simulink model "STDiscovery"  (R2017b)
settings: Solver=FixedStepAuto  StartTime=0.0  StopTime=0.01  FixedStep=Abtastzeit  RelTol=1e-3
PreLoadFcn:
  | waijung.modelPreload; % Required for working with Waijung Blockset. Do not remove.
model workspace (MAT data in the model file):
  Abtastzeit = 0.01
  Servo_IN_min = 0.894
  SimulationDutyCycle = 27
undefined symbols (not defined in the file): HSEOSC, Link, LQFP176, ST, Statusbits, Steuerbits, STM32F417IG
libraries: simulink x17, stm32f4_io_lib x16, simulink_extras x8, stm32f4_adc_lib x7, powerlib_meascontrol x4, stm32f4_device_config_lib x1
(part 4 of 4)

== system STDiscovery/Aktorik/Ansteuerung Motor/Skaliere PWM Ausgang wieder in wert zwischen( + -100) zum Loggen  ==
  note: in muss immer mit kleinstem wert anfangen
  note: 100(Gas)
      | -100(Rückwärts)
  note: %
  Wert in % für 50Hz PWM : Inport
  Constant1 : Constant  Value=100
  Constant2 : Constant  Value=0
  Constant3 : Constant  Value=-100
  Constant4 : Constant  Value=5.5
  Constant5 : Constant  Value=7.45
  Constant6 : Constant  Value=9.5
  Skaliere lN nach OUT : Subsystem
  "Wert zwischen 100 und -100 " : Outport
  wires:
  Skaliere lN nach OUT/1(OUT_SIGNAL) -> "Wert zwischen 100 und -100 "/1
  Wert in % für 50Hz PWM/1 -> Skaliere lN nach OUT/1(IN_SIGNAL)
  Constant1/1 -> Skaliere lN nach OUT/5(OUT_min)
  Constant2/1 -> Skaliere lN nach OUT/6(OUT_mitte)
  Constant3/1 -> Skaliere lN nach OUT/7(OUT_max)
  Constant6/1 -> Skaliere lN nach OUT/4(IN_max)
  Constant5/1 -> Skaliere lN nach OUT/3(IN_mitte)
  Constant4/1 -> Skaliere lN nach OUT/2(IN_min)

== system STDiscovery/Aktorik/Ansteuerung Servo/Logik  ==
  Fernbedienung Signal : Inport
  Moduswahl (1=autonom 0=manuell) : Inport  Port=2
  Jetson Signal : Inport  Port=3
  "(Einschaltverzögerung) Wartezeit Anhalten Erst 1s aktuellen autonomen Lenkeinschlag halten, dann Fernbedienung übernehmen " : powerlib_meascontrol/Logic/On Delay  DelayType=On delay  delay=1  ic=1  Ts=0
      settings: SourceProductName=Simscape Power Systems
  Data Type Conversion : DataTypeConversion  OutDataTypeStr=double
  "Erst 1s aktuellen autonomen Lenkeinschlag halten, dann Fernbedienung übernehmen" : Switch  Criteria=u2 > Threshold
  Modus Auswahl : Switch  Criteria=u2 > Threshold
  Output Pin : Outport
  wires:
  Data Type Conversion/1 -> "Erst 1s aktuellen autonomen Lenkeinschlag halten, dann Fernbedienung übernehmen"/3  "manuell"
  Moduswahl (1=autonom 0=manuell)/1 -> "(Einschaltverzögerung) Wartezeit Anhalten Erst 1s aktuellen autonomen Lenkeinschlag halten, dann Fernbedienung übernehmen "/1, Modus Auswahl/2
  Modus Auswahl/1 -> Output Pin/1  "Ausgang zum servo"
  "Erst 1s aktuellen autonomen Lenkeinschlag halten, dann Fernbedienung übernehmen"/1 -> Modus Auswahl/3  "manuell"
  Jetson Signal/1 -> Modus Auswahl/1, "Erst 1s aktuellen autonomen Lenkeinschlag halten, dann Fernbedienung übernehmen"/1  "autonom"
  "(Einschaltverzögerung) Wartezeit Anhalten Erst 1s aktuellen autonomen Lenkeinschlag halten, dann Fernbedienung übernehmen "/1 -> "Erst 1s aktuellen autonomen Lenkeinschlag halten, dann Fernbedienung übernehmen"/2
  Fernbedienung Signal/1 -> Data Type Conversion/1

== system STDiscovery/Aktorik/Ansteuerung Servo/Plausibilitäts Check ==
  In1 : Inport
  "Gib Mittelstellung aus, wenn mit Signal etwas nicht Stimmt" : Switch  Criteria=u2 > Threshold
  Logical Operator : Logic  AllPortsSameDT=off  OutDataTypeStr=boolean
  Mittelstellung : Constant  Value=0.001407
  Relational Operator : RelationalOperator  Operator=<  OutDataTypeStr=boolean  RndMeth=Nearest
  Relational Operator1 : RelationalOperator  Operator=>  OutDataTypeStr=boolean  RndMeth=Nearest
  "ok max " : Constant  Value=0.0021
  ok min : Constant  Value=0.0008
  Out1 : Outport
  wires:
  In1/1 -> Relational Operator1/1, Relational Operator/1, "Gib Mittelstellung aus, wenn mit Signal etwas nicht Stimmt"/1
  Logical Operator/1 -> "Gib Mittelstellung aus, wenn mit Signal etwas nicht Stimmt"/2
  "Gib Mittelstellung aus, wenn mit Signal etwas nicht Stimmt"/1 -> Out1/1
  Mittelstellung/1 -> "Gib Mittelstellung aus, wenn mit Signal etwas nicht Stimmt"/3
  Relational Operator1/1 -> Logical Operator/2
  Relational Operator/1 -> Logical Operator/1
  ok min/1 -> Relational Operator1/2
  "ok max "/1 -> Relational Operator/2

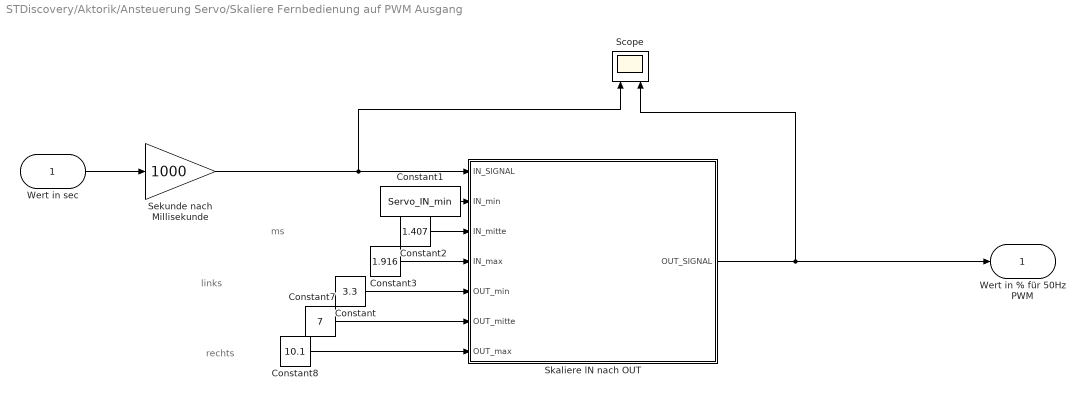
== system STDiscovery/Aktorik/Ansteuerung Servo/Skaliere Fernbedienung auf PWM Ausgang ==
  note: ms
  note: links
  note: rechts
  Wert in sec : Inport
  Constant : Constant  Value=3.3
  Constant1 : Constant  Value=Servo_IN_min
  Constant2 : Constant  Value=1.407
  Constant3 : Constant  Value=1.916
  Constant7 : Constant  Value=7
  Constant8 : Constant  Value=10.1
  Scope : Scope  NumInputPorts=2
  Sekunde nach Millisekunde : Gain  Gain=1000
  Skaliere lN nach OUT : Subsystem
  Wert in % für 50Hz PWM : Outport
  wires:
  Constant/1 -> Skaliere lN nach OUT/5(OUT_min)
  Wert in sec/1 -> Sekunde nach Millisekunde/1
  Skaliere lN nach OUT/1(OUT_SIGNAL) -> Scope/2, Wert in % für 50Hz PWM/1
  Constant3/1 -> Skaliere lN nach OUT/4(IN_max)
  Constant2/1 -> Skaliere lN nach OUT/3(IN_mitte)
  Constant1/1 -> Skaliere lN nach OUT/2(IN_min)
  Sekunde nach Millisekunde/1 -> Scope/1, Skaliere lN nach OUT/1(IN_SIGNAL)
  Constant7/1 -> Skaliere lN nach OUT/6(OUT_mitte)
  Constant8/1 -> Skaliere lN nach OUT/7(OUT_max)

== system STDiscovery/Aktorik/Ansteuerung Servo/Skaliere Stellwinkel auf PWM Ausgang ==
  note: Stellwinkel
  note: rechts
  note: links
  Stellwinkel : Inport
  Constant : Constant  Value=3.3
  Constant1 : Constant  Value=-25
  Constant2 : Constant  Value=0
  Constant3 : Constant  Value=25
  Constant7 : Constant  Value=7
  Constant8 : Constant  Value=10.1
  Skaliere lN nach OUT : Subsystem
  Wert in % für 50Hz PWM : Outport
  wires:
  Constant/1 -> Skaliere lN nach OUT/5(OUT_min)
  Skaliere lN nach OUT/1(OUT_SIGNAL) -> Wert in % für 50Hz PWM/1
  Constant3/1 -> Skaliere lN nach OUT/4(IN_max)
  Constant2/1 -> Skaliere lN nach OUT/3(IN_mitte)
  Constant1/1 -> Skaliere lN nach OUT/2(IN_min)
  Stellwinkel/1 -> Skaliere lN nach OUT/1(IN_SIGNAL)
  Constant8/1 -> Skaliere lN nach OUT/7(OUT_max)
  Constant7/1 -> Skaliere lN nach OUT/6(OUT_mitte)

== system STDiscovery/Aktorik/Ansteuerung Servo/Skaliere steuer Stellwinkel wieder in Grad zum Loggen ==
  note: rechts
  note: links
  note: Stellwinkel
  Wert in % für 50Hz PWM : Inport
  Constant : Constant  Value=3.3
  Constant1 : Constant  Value=-25
  Constant2 : Constant  Value=0
  Constant3 : Constant  Value=25
  Constant7 : Constant  Value=7
  Constant8 : Constant  Value=10.1
  Skaliere lN nach OUT : Subsystem
  Stellwinkel : Outport
  wires:
  Skaliere lN nach OUT/1(OUT_SIGNAL) -> Stellwinkel/1
  Constant/1 -> Skaliere lN nach OUT/2(IN_min)
  Wert in % für 50Hz PWM/1 -> Skaliere lN nach OUT/1(IN_SIGNAL)
  Constant7/1 -> Skaliere lN nach OUT/3(IN_mitte)
  Constant8/1 -> Skaliere lN nach OUT/4(IN_max)
  Constant2/1 -> Skaliere lN nach OUT/6(OUT_mitte)
  Constant3/1 -> Skaliere lN nach OUT/7(OUT_max)
  Constant1/1 -> Skaliere lN nach OUT/5(OUT_min)

== system STDiscovery/Aktorik/Modusauswahl Autonom oder Manuell Ueberwachung ob Eingriff durch Fernbedienung/Motor Überwachung Eingriff durch Fernbedienung? ==
  Dutycycle in % : Inport
  Betrag bilden für negative Abweichunge : Abs
  Ist die Aktuelle Abweichung größer als die Maximal erlaubte? : RelationalOperator  Operator=>  OutDataTypeStr=boolean  RndMeth=Nearest
  Maximale Abweichung : Constant  Value=0.2
  "Mittelwert, in % wenn Fernsteuerung in der Mitte steht" : Constant  Value=7.45
  Subtract : Sum  Inputs=|+-
  Ja/Nein : Outport
  wires:
  "Mittelwert, in % wenn Fernsteuerung in der Mitte steht"/1 -> Subtract/2
  Betrag bilden für negative Abweichunge/1 -> Ist die Aktuelle Abweichung größer als die Maximal erlaubte?/1
  Maximale Abweichung/1 -> Ist die Aktuelle Abweichung größer als die Maximal erlaubte?/2
  Dutycycle in %/1 -> Subtract/1
  Subtract/1 -> Betrag bilden für negative Abweichunge/1
  Ist die Aktuelle Abweichung größer als die Maximal erlaubte?/1 -> Ja/Nein/1

== system STDiscovery/Aktorik/Modusauswahl Autonom oder Manuell Ueberwachung ob Eingriff durch Fernbedienung/Servo Überwachung Eingriff durch Fernbedienung? ==
  Dutycycle in % : Inport
  Betrag bilden für negative Abweichungen : Abs
  Ist die aktuelle Abweichung größer als die maximal erlaubte? : RelationalOperator  Operator=>  OutDataTypeStr=boolean  RndMeth=Nearest
  Maximale Abweichung : Constant  Value=0.2
  "Mittelwert, in % wenn Fernsteuerung in der Mitte steht" : Constant  Value=7
  Subtract : Sum  Inputs=|+-
  Ja/Nein : Outport
  wires:
  "Mittelwert, in % wenn Fernsteuerung in der Mitte steht"/1 -> Subtract/2
  Betrag bilden für negative Abweichungen/1 -> Ist die aktuelle Abweichung größer als die maximal erlaubte?/1
  Maximale Abweichung/1 -> Ist die aktuelle Abweichung größer als die maximal erlaubte?/2
  Dutycycle in %/1 -> Subtract/1
  Subtract/1 -> Betrag bilden für negative Abweichungen/1
  Ist die aktuelle Abweichung größer als die maximal erlaubte?/1 -> Ja/Nein/1

== system STDiscovery/Debug/Subsystem/Safety 2.5 |<--->|12.5 ==
  In1 : Inport
  Constant : Constant  Value=2.5
  Constant1 : Constant  Value=12.5
  Data Type Conversion : DataTypeConversion
  Data Type Conversion1 : DataTypeConversion
  Switch : Switch  Criteria=u2 > Threshold  Threshold=2.5
  Switch1 : Switch  Criteria=u2 > Threshold  Threshold=12.5
  Out1 : Outport
  wires:
  Switch/1 -> Switch1/3, Switch1/2
  In1/1 -> Switch/1, Switch/2
  Switch1/1 -> Out1/1
  Constant/1 -> Data Type Conversion/1
  Constant1/1 -> Data Type Conversion1/1
  Data Type Conversion1/1 -> Switch1/1
  Data Type Conversion/1 -> Switch/3

== system STDiscovery/Debug/Subsystem1/Safety 2.5 |<--->|12.5 ==
  In1 : Inport
  Constant : Constant  Value=2.5
  Constant1 : Constant  Value=12.5
  Data Type Conversion : DataTypeConversion
  Data Type Conversion1 : DataTypeConversion
  Switch : Switch  Criteria=u2 > Threshold  Threshold=2.5
  Switch1 : Switch  Criteria=u2 > Threshold  Threshold=12.5
  Out1 : Outport
  wires:
  Switch/1 -> Switch1/3, Switch1/2
  In1/1 -> Switch/1, Switch/2
  Switch1/1 -> Out1/1
  Constant/1 -> Data Type Conversion/1
  Constant1/1 -> Data Type Conversion1/1
  Data Type Conversion1/1 -> Switch1/1
  Data Type Conversion/1 -> Switch/3

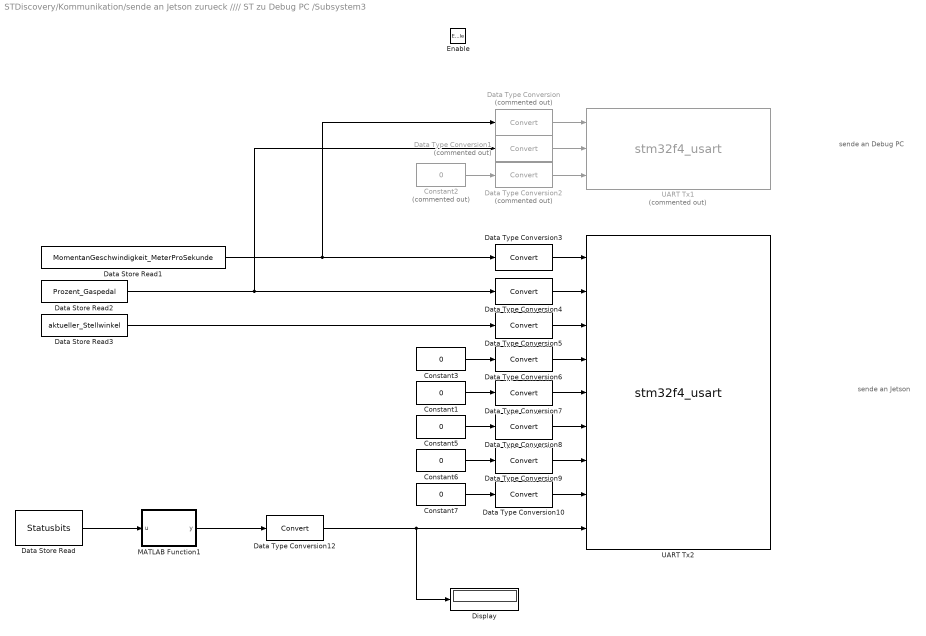
== system STDiscovery/Kommunikation/sende an Jetson zurueck //// ST zu Debug PC /Subsystem3 ==
  note: sende an Debug PC
  note: sende an Jetson
  Enable : EnablePort
  Constant{1,3,5..7} (5 alike) : Constant  Value=0
  Constant2 : Constant  Commented=on  Value=0
  Data Store Read : DataStoreRead  DataStoreName=Statusbits
  Data Store Read1 : DataStoreRead  DataStoreName=MomentanGeschwindigkeit_MeterProSekunde
  Data Store Read2 : DataStoreRead  DataStoreName=Prozent_Gaspedal
  Data Store Read3 : DataStoreRead  DataStoreName=aktueller_Stellwinkel
  Data Type Conversion : DataTypeConversion  Commented=on
  Data Type Conversion1 : DataTypeConversion  Commented=on
  Data Type Conversion{3..10,12} (9 alike) : DataTypeConversion
  Data Type Conversion2 : DataTypeConversion  Commented=on
  Display : Display
  MATLAB Function1 : MATLAB Function  TreatAsAtomicUnit=on
  UART Tx1 : S-Function  Priority=1  Commented=on  FunctionName=stm32f4_usart  Parameters=configuration,uartmodule,transfer,baudrate,inputtype,outputtype,confstr,binheaderarray,binterminatorarray,asciiheader,asciiterminator,bindatalength,packetmode,varname,sampletime,sampletimestr,blockid  SFunctionDeploymentMode=off  EnableBusSupport=off  mask(stm32f4_usart){configuration=Tx, uartmodule=3, baudrate=115200, databits=8, parity=No, stopbit=1, remaptxpin=Not used, remaprxpin=Not used, flowcontrol=None, remapctspin=Not used, remaprtspin=Not used, advanceoptions=off, rxbuffersize=512, txbuffersize=512, transfer=Blocking, packetmode=Ascii, binheader='7E 7E', binterminator='03 03', porttype_double=1, porttype_single=0, porttype_int8=1, porttype_uint8=0, porttype_int16=0, porttype_uint16=0, porttype_int32=0, porttype_uint32=0, asciiformat='Antwort von ST:    Momentangeschwindigkeit: %f   , Hz: %f   ,TEST:  %f', rx_asciiterminator=CRLF (0x0D 0x0A - "\r\n"), tx_asciiterminator=CRLF (0x0D 0x0A - "\r\n"), storagename=S, varname=, inputtype=[3  1 1 1], outputtype=[0], binheaderarray=[0], binterminatorarray=[0], bindatalength=0, asciiheader='Antwort von ST:    Momentangeschwindigkeit: %f   , Hz: %f   ,TEST:  %f\r\n', asciiterminator=[2 13 10], sampletime=-1, sampletimestr=-1, blockid=KommunikationsendeanJetsonzurueckSTzuDebugPCSubsystem3UARTTx1, confstr=[ "dummy", "0", "*", "*", "0", "*", "*", "0", "*", "*", "0", "*", "*", "1", "4", "3", "1", "4", "1", "512", "512", "1", "3", "115200", "8", "No", "1", "None", "USART3"], lastmodule=1}
      mask prompts: uartmodule "UART Module"; baudrate "Baud rate (bps)"; databits "Data bits"; stopbit "Stop bit"; remaptxpin "Tx Pin"; remaprxpin "Rx Pin"; flowcontrol "Hardware flow control"; remapctspin "HW Flow control, CTS Pin"; remaprtspin "HW Flow control, RTS Pin"; advanceoptions "Advance options"; rxbuffersize "Rx buffer size (bytes)"; txbuffersize "Tx buffer size (bytes)"; packetmode "Packet mode"; binheader "Binary header (example: '7E 7E')"; binterminator "Binary terminator (example: '03 03')"; porttype_double "Number of data port, type DOUBLE"; porttype_single "Number of data port, type SINGLE"; porttype_int8 "Number of data port, type INT8"; porttype_uint8 "Number of data port, type UINT8"; porttype_int16 "Number of data port, type INT16"; porttype_uint16 "Number of data port, type UINT16"; porttype_int32 "Number of data port, type INT32"; porttype_uint32 "Number of data port, type UINT32"; asciiformat "Ascii format"; rx_asciiterminator "End of packet"; tx_asciiterminator "End of packet"; storagename "Buffer"; varname "Var name"; inputtype "Input data type"; outputtype "Output data type"; binheaderarray "Binary header"; binterminatorarray "Binary terminator"; bindatalength "Binary data length"; asciiheader "Ascii header (printf format)"; asciiterminator "Ascii terminator"; sampletime "Sample time (sec)"; sampletimestr "Compiled sample time (sec) in string"; confstr "Configuration string"; lastmodule "Last module selected"
      mask help:
      | Data type for Ascii format
      | %u, %i, %d, %o, %x: uint32
      | %e, %g, %f: single
      | %c: int8
      mask init:
      | stm32f4_usart_callback('init');
      mask Help: web(fullfile(waijungdocroot,'stm32f4_usart_tx.htm'), '-browser')
      mask TypeOptions configuration: Setup | Tx | Rx
      mask Callback configuration: stm32f4_usart_callback('configuration');
      mask TypeOptions uartmodule: 1 | 2 | 3 | 4 | 5 | 6
      mask Callback uartmodule: stm32f4_usart_callback('uartmodule');
      mask Callback baudrate: stm32f4_usart_callback('baudrate');
      mask TypeOptions databits: 8
      mask TypeOptions parity: No | Odd | Even
      mask TypeOptions stopbit: 0.5 | 1 | 1.5 | 2
      mask TypeOptions remaptxpin: Not used | A9 | B6
      mask TypeOptions remaprxpin: Not used | A10 | B7
      mask TypeOptions flowcontrol: None | RTS | CTS | RTS/CTS
      mask Callback flowcontrol: stm32f4_usart_callback('flowcontrol');
      mask TypeOptions remapctspin: Not used | A11
      mask TypeOptions remaprtspin: Not used | A12
      mask Callback advanceoptions: stm32f4_usart_callback('advanceoptions');
      mask TypeOptions rxbuffersize: 16 | 32 | 64 | 128 | 256 | 512 | 1024 | 2048
      mask TypeOptions txbuffersize: 16 | 32 | 64 | 128 | 256 | 512 | 1024 | 2048
      mask TypeOptions transfer: Blocking | Non-Blocking
      mask Callback transfer: stm32f4_usart_callback('transfer');
      mask TypeOptions packetmode: Ascii | Binary | String Buffer
      mask Callback packetmode: stm32f4_usart_callback('packetmode');
      mask Callback binheader: stm32f4_usart_callback('binheader');
      mask Callback binterminator: stm32f4_usart_callback('binterminator');
      mask Callback porttype_double: stm32f4_usart_callback('porttype');
      mask Callback porttype_single: stm32f4_usart_callback('porttype');
      mask Callback porttype_int8: stm32f4_usart_callback('porttype');
      mask Callback porttype_uint8: stm32f4_usart_callback('porttype');
      mask Callback porttype_int16: stm32f4_usart_callback('porttype');
      mask Callback porttype_uint16: stm32f4_usart_callback('porttype');
      mask Callback porttype_int32: stm32f4_usart_callback('porttype');
      mask Callback porttype_uint32: stm32f4_usart_callback('porttype');
      mask Callback asciiformat: stm32f4_usart_callback('asciiformat');
      mask TypeOptions rx_asciiterminator: CR (0x0D - "\r") | LF (0x0A - "\n") | CRLF (0x0D 0x0A - "\r\n")
      mask Callback rx_asciiterminator: stm32f4_usart_callback('rx_asciiterminator');
      mask TypeOptions tx_asciiterminator: CR (0x0D - "\r") | LF (0x0A - "\n") | CRLF (0x0D 0x0A - "\r\n") | None
      mask Callback tx_asciiterminator: stm32f4_usart_callback('tx_asciiterminator');
      mask TypeOptions storagename: <Please insert a storage name> | S
      mask Callback storagename: stm32f4_usart_callback('storagename');
      mask Callback varname: stm32f4_usart_callback('varname');
      mask Callback sampletime: stm32f4_usart_callback('sampletime');
      mask Callback sampletimestr: stm32f4_usart_callback('sampletimestr');
      mask Callback blockid: stm32f4_usart_callback('blockid');
      mask Display: text(0.95, 0.5, 'Module: USART3_Tx\nPacket: Ascii\nTransfer: Blocking\nTs (sec): -1','ver','middle','hor','right'); port_label('input', 1,'single'); port_label('input', 2,'single'); port_label('input', 3,'single');
  UART Tx2 : S-Function  Priority=1  FunctionName=stm32f4_usart  Parameters=configuration,uartmodule,transfer,baudrate,inputtype,outputtype,confstr,binheaderarray,binterminatorarray,asciiheader,asciiterminator,bindatalength,packetmode,varname,sampletime,sampletimestr,blockid  SFunctionDeploymentMode=off  EnableBusSupport=off  mask(stm32f4_usart){configuration=Tx, uartmodule=1, baudrate=115200, databits=8, parity=No, stopbit=1, remaptxpin=Not used, remaprxpin=Not used, flowcontrol=None, remapctspin=Not used, remaprtspin=Not used, advanceoptions=off, rxbuffersize=512, txbuffersize=512, transfer=Blocking, packetmode=Binary, binheader='', binterminator='', porttype_double=0, porttype_single=8, porttype_int8=0, porttype_uint8=0, porttype_int16=0, porttype_uint16=1, porttype_int32=0, porttype_uint32=0, asciiformat='Antwort von ST:  %f', rx_asciiterminator=CRLF (0x0D 0x0A - "\r\n"), tx_asciiterminator=CRLF (0x0D 0x0A - "\r\n"), storagename=S, varname=, inputtype=[9  1 1 1 1 1 1 1 1 5], outputtype=[0], binheaderarray=[0 ], binterminatorarray=[0 ], bindatalength=34, asciiheader='Antwort von ST:  %f\r\n', asciiterminator=[2 13 10], sampletime=-1, sampletimestr=-1, blockid=KommunikationsendeanJetsonzurueckSTzuDebugPCSubsystem3UARTTx2, confstr=[ "dummy", "0", "*", "*", "0", "*", "*", "0", "*", "*", "0", "*", "*", "2", "4", "7", "2", "4", "2", "512", "512", "2", "1", "115200", "8", "No", "1", "None", "USART1"], lastmodule=1}
      mask prompts: uartmodule "UART Module"; baudrate "Baud rate (bps)"; databits "Data bits"; stopbit "Stop bit"; remaptxpin "Tx Pin"; remaprxpin "Rx Pin"; flowcontrol "Hardware flow control"; remapctspin "HW Flow control, CTS Pin"; remaprtspin "HW Flow control, RTS Pin"; advanceoptions "Advance options"; rxbuffersize "Rx buffer size (bytes)"; txbuffersize "Tx buffer size (bytes)"; packetmode "Packet mode"; binheader "Binary header (example: '7E 7E')"; binterminator "Binary terminator (example: '03 03')"; porttype_double "Number of data port, type DOUBLE"; porttype_single "Number of data port, type SINGLE"; porttype_int8 "Number of data port, type INT8"; porttype_uint8 "Number of data port, type UINT8"; porttype_int16 "Number of data port, type INT16"; porttype_uint16 "Number of data port, type UINT16"; porttype_int32 "Number of data port, type INT32"; porttype_uint32 "Number of data port, type UINT32"; asciiformat "Ascii format"; rx_asciiterminator "End of packet"; tx_asciiterminator "End of packet"; storagename "Buffer"; varname "Var name"; inputtype "Input data type"; outputtype "Output data type"; binheaderarray "Binary header"; binterminatorarray "Binary terminator"; bindatalength "Binary data length"; asciiheader "Ascii header (printf format)"; asciiterminator "Ascii terminator"; sampletime "Sample time (sec)"; sampletimestr "Compiled sample time (sec) in string"; confstr "Configuration string"; lastmodule "Last module selected"
      mask help:
      | Data type for Ascii format
      | %u, %i, %d, %o, %x: uint32
      | %e, %g, %f: single
      | %c: int8
      mask init:
      | stm32f4_usart_callback('init');
      mask Help: web(fullfile(waijungdocroot,'stm32f4_usart_tx.htm'), '-browser')
      mask TypeOptions configuration: Setup | Tx | Rx
      mask Callback configuration: stm32f4_usart_callback('configuration');
      mask TypeOptions uartmodule: 1 | 2 | 3 | 4 | 5 | 6
      mask Callback uartmodule: stm32f4_usart_callback('uartmodule');
      mask Callback baudrate: stm32f4_usart_callback('baudrate');
      mask TypeOptions databits: 8
      mask TypeOptions parity: No | Odd | Even
      mask TypeOptions stopbit: 0.5 | 1 | 1.5 | 2
      mask TypeOptions remaptxpin: Not used | A9 | B6
      mask TypeOptions remaprxpin: Not used | A10 | B7
      mask TypeOptions flowcontrol: None | RTS | CTS | RTS/CTS
      mask Callback flowcontrol: stm32f4_usart_callback('flowcontrol');
      mask TypeOptions remapctspin: Not used | A11
      mask TypeOptions remaprtspin: Not used | A12
      mask Callback advanceoptions: stm32f4_usart_callback('advanceoptions');
      mask TypeOptions rxbuffersize: 16 | 32 | 64 | 128 | 256 | 512 | 1024 | 2048
      mask TypeOptions txbuffersize: 16 | 32 | 64 | 128 | 256 | 512 | 1024 | 2048
      mask TypeOptions transfer: Blocking | Non-Blocking
      mask Callback transfer: stm32f4_usart_callback('transfer');
      mask TypeOptions packetmode: Ascii | Binary | String Buffer
      mask Callback packetmode: stm32f4_usart_callback('packetmode');
      mask Callback binheader: stm32f4_usart_callback('binheader');
      mask Callback binterminator: stm32f4_usart_callback('binterminator');
      mask Callback porttype_double: stm32f4_usart_callback('porttype');
      mask Callback porttype_single: stm32f4_usart_callback('porttype');
      mask Callback porttype_int8: stm32f4_usart_callback('porttype');
      mask Callback porttype_uint8: stm32f4_usart_callback('porttype');
      mask Callback porttype_int16: stm32f4_usart_callback('porttype');
      mask Callback porttype_uint16: stm32f4_usart_callback('porttype');
      mask Callback porttype_int32: stm32f4_usart_callback('porttype');
      mask Callback porttype_uint32: stm32f4_usart_callback('porttype');
      mask Callback asciiformat: stm32f4_usart_callback('asciiformat');
      mask TypeOptions rx_asciiterminator: CR (0x0D - "\r") | LF (0x0A - "\n") | CRLF (0x0D 0x0A - "\r\n")
      mask Callback rx_asciiterminator: stm32f4_usart_callback('rx_asciiterminator');
      mask TypeOptions tx_asciiterminator: CR (0x0D - "\r") | LF (0x0A - "\n") | CRLF (0x0D 0x0A - "\r\n") | None
      mask Callback tx_asciiterminator: stm32f4_usart_callback('tx_asciiterminator');
      mask TypeOptions storagename: <Please insert a storage name> | S
      mask Callback storagename: stm32f4_usart_callback('storagename');
      mask Callback varname: stm32f4_usart_callback('varname');
      mask Callback sampletime: stm32f4_usart_callback('sampletime');
      mask Callback sampletimestr: stm32f4_usart_callback('sampletimestr');
      mask Callback blockid: stm32f4_usart_callback('blockid');
      mask Display: text(0.95, 0.5, 'Module: USART1_Tx\nPacket: Binary\nTransfer: Blocking\nTs (sec): -1','ver','middle','hor','right'); port_label('input', 1,'single'); port_label('input', 2,'single'); port_label('input', 3,'single'); port_label('input', 4,'single'); port_label('input', 5,'single'); port_label('input', 6,'single'); port_label('input', 7,'single'); port_label('input', 8,'single'); port_label('input', 9,'uint16');
  wires:
  Data Type Conversion/1 -> UART Tx1/1
  Data Type Conversion2/1 -> UART Tx1/3
  Data Type Conversion1/1 -> UART Tx1/2
  Constant2/1 -> Data Type Conversion2/1
  Data Store Read1/1 -> Data Type Conversion/1, Data Type Conversion3/1
  Data Type Conversion3/1 -> UART Tx2/1
  Data Store Read2/1 -> Data Type Conversion1/1, Data Type Conversion4/1
  Data Type Conversion4/1 -> UART Tx2/2
  Data Type Conversion5/1 -> UART Tx2/3
  Data Store Read3/1 -> Data Type Conversion5/1
  Constant3/1 -> Data Type Conversion6/1
  Data Type Conversion6/1 -> UART Tx2/4
  Data Type Conversion7/1 -> UART Tx2/5
  Constant1/1 -> Data Type Conversion7/1
  Constant5/1 -> Data Type Conversion8/1
  Data Type Conversion8/1 -> UART Tx2/6
  Constant6/1 -> Data Type Conversion9/1
  Data Type Conversion9/1 -> UART Tx2/7
  Constant7/1 -> Data Type Conversion10/1
  Data Type Conversion10/1 -> UART Tx2/8
  MATLAB Function1/1(y) -> Data Type Conversion12/1
  Data Store Read/1 -> MATLAB Function1/1(u)
  Data Type Conversion12/1 -> Display/1, UART Tx2/9

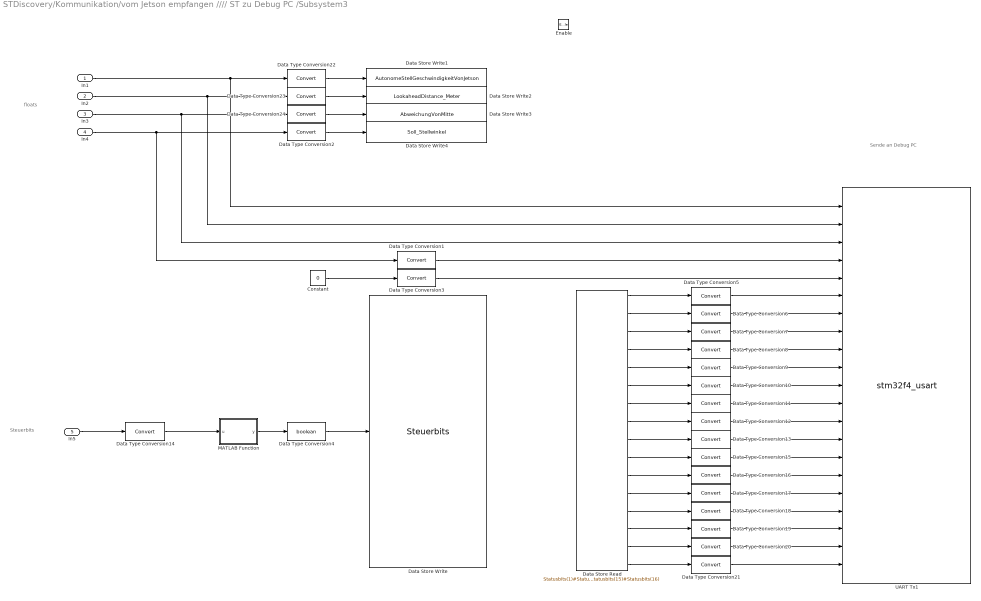
== system STDiscovery/Kommunikation/vom Jetson empfangen //// ST zu Debug PC /Subsystem3 ==
  note: floats
  note: Sende an Debug PC
  note: Steuerbits
  In1 : Inport
  In2 : Inport  Port=2
  In3 : Inport  Port=3
  In4 : Inport  Port=4
  In5 : Inport  Port=5
  Enable : EnablePort
  Constant : Constant  Value=0
  Data Store Read : DataStoreRead  DataStoreName=Statusbits  DataStoreElements=Statusbits(1)#Statusbits(2)#Statusbits(3)#Statusbits(4)#Statusbits(5)#Statusbits(6)#Statusbits(7)#Statusbits(8)#Statusbits(9)#Statusbits(10)#Statusbits(11)#Statusbits(12)#Statusbits(13)#Statusbits(14)#Statusbits(15)#Statusbits(16)
  Data Store Write : DataStoreWrite  DataStoreName=Steuerbits
  Data Store Write1 : DataStoreWrite  DataStoreName=AutonomeStellGeschwindigkeitVonJetson
  Data Store Write2 : DataStoreWrite  DataStoreName=LookaheadDistance_Meter
  Data Store Write3 : DataStoreWrite  DataStoreName=AbweichungVonMitte
  Data Store Write4 : DataStoreWrite  DataStoreName=Soll_Stellwinkel
  Data Type Conversion{1..3,5..24} (23 alike) : DataTypeConversion
  Data Type Conversion4 : DataTypeConversion  OutDataTypeStr=boolean
  MATLAB Function : MATLAB Function  TreatAsAtomicUnit=on
  UART Tx1 : S-Function  Priority=1  FunctionName=stm32f4_usart  Parameters=configuration,uartmodule,transfer,baudrate,inputtype,outputtype,confstr,binheaderarray,binterminatorarray,asciiheader,asciiterminator,bindatalength,packetmode,varname,sampletime,sampletimestr,blockid  SFunctionDeploymentMode=off  EnableBusSupport=off  mask(stm32f4_usart){configuration=Tx, uartmodule=3, baudrate=115200, databits=8, parity=No, stopbit=1, remaptxpin=Not used, remaprxpin=Not used, flowcontrol=None, remapctspin=Not used, remaprtspin=Not used, advanceoptions=off, rxbuffersize=512, txbuffersize=512, transfer=Blocking, packetmode=Ascii, binheader='7E 7E', binterminator='03 03', porttype_double=1, porttype_single=0, porttype_int8=1, porttype_uint8=0, porttype_int16=0, porttype_uint16=0, porttype_int32=0, porttype_uint32=0, asciiformat=' Geschwindigkeit: %f   ,Lookahead:  %f , Deltax: %f  , Reserve: %f  ,\n Winkel:%f \n (1): %f \n (2): %f \n (3): %f \n (4): %f \n (5): %f \n (6): %f \n (7): %f \n (8): %f \n (9): %f \n (10): %f \n (11): %f \n (12): %f \n (13): %f \n (14): %f \n (15): %f \n (16): %f', rx_asciiterminator=CRLF (0x0D 0x0A - "\r\n"), tx_asciiterminator=CRLF (0x0D 0x0A - "\r\n"), storagename=S, varname=, inputtype=[21  1 1 1 1 1 1 1 1 1 1 1 1 1 1 1 1 1 1 1 1 1], outputtype=[0], binheaderarray=[0], binterminatorarray=[0], bindatalength=0, asciiheader=' Geschwindigkeit: %f   ,Lookahead:  %f , Deltax: %f  , Reserve: %f  ,\n Winkel:%f \n (1): %f \n (2): %f \n (3): %f \n (4): %f \n (5): %f \n (6): %f \n (7): %f \n (8): %f \n (9): %f \n (10): %f \n (11): %f \n (12): %f \n (13): %f \n (14): %f \n (15): %f \n (16): %f\r\n', asciiterminator=[2 13 10], sampletime=0.1, sampletimestr=-1, blockid=KommunikationvomJetsonempfangenSTzuDebugPCSubsystem3UARTTx1, confstr=[ "dummy", "0", "*", "*", "0", "*", "*", "0", "*", "*", "0", "*", "*", "1", "4", "3", "1", "4", "1", "512", "512", "1", "3", "115200", "8", "No", "1", "None", "USART3"], lastmodule=1}
      mask prompts: uartmodule "UART Module"; baudrate "Baud rate (bps)"; databits "Data bits"; stopbit "Stop bit"; remaptxpin "Tx Pin"; remaprxpin "Rx Pin"; flowcontrol "Hardware flow control"; remapctspin "HW Flow control, CTS Pin"; remaprtspin "HW Flow control, RTS Pin"; advanceoptions "Advance options"; rxbuffersize "Rx buffer size (bytes)"; txbuffersize "Tx buffer size (bytes)"; packetmode "Packet mode"; binheader "Binary header (example: '7E 7E')"; binterminator "Binary terminator (example: '03 03')"; porttype_double "Number of data port, type DOUBLE"; porttype_single "Number of data port, type SINGLE"; porttype_int8 "Number of data port, type INT8"; porttype_uint8 "Number of data port, type UINT8"; porttype_int16 "Number of data port, type INT16"; porttype_uint16 "Number of data port, type UINT16"; porttype_int32 "Number of data port, type INT32"; porttype_uint32 "Number of data port, type UINT32"; asciiformat "Ascii format"; rx_asciiterminator "End of packet"; tx_asciiterminator "End of packet"; storagename "Buffer"; varname "Var name"; inputtype "Input data type"; outputtype "Output data type"; binheaderarray "Binary header"; binterminatorarray "Binary terminator"; bindatalength "Binary data length"; asciiheader "Ascii header (printf format)"; asciiterminator "Ascii terminator"; sampletime "Sample time (sec)"; sampletimestr "Compiled sample time (sec) in string"; confstr "Configuration string"; lastmodule "Last module selected"
      mask help:
      | Data type for Ascii format
      | %u, %i, %d, %o, %x: uint32
      | %e, %g, %f: single
      | %c: int8
      mask init:
      | stm32f4_usart_callback('init');
      mask Help: web(fullfile(waijungdocroot,'stm32f4_usart_tx.htm'), '-browser')
      mask TypeOptions configuration: Setup | Tx | Rx
      mask Callback configuration: stm32f4_usart_callback('configuration');
      mask TypeOptions uartmodule: 1 | 2 | 3 | 4 | 5 | 6
      mask Callback uartmodule: stm32f4_usart_callback('uartmodule');
      mask Callback baudrate: stm32f4_usart_callback('baudrate');
      mask TypeOptions databits: 8
      mask TypeOptions parity: No | Odd | Even
      mask TypeOptions stopbit: 0.5 | 1 | 1.5 | 2
      mask TypeOptions remaptxpin: Not used | A9 | B6
      mask TypeOptions remaprxpin: Not used | A10 | B7
      mask TypeOptions flowcontrol: None | RTS | CTS | RTS/CTS
      mask Callback flowcontrol: stm32f4_usart_callback('flowcontrol');
      mask TypeOptions remapctspin: Not used | A11
      mask TypeOptions remaprtspin: Not used | A12
      mask Callback advanceoptions: stm32f4_usart_callback('advanceoptions');
      mask TypeOptions rxbuffersize: 16 | 32 | 64 | 128 | 256 | 512 | 1024 | 2048
      mask TypeOptions txbuffersize: 16 | 32 | 64 | 128 | 256 | 512 | 1024 | 2048
      mask TypeOptions transfer: Blocking | Non-Blocking
      mask Callback transfer: stm32f4_usart_callback('transfer');
      mask TypeOptions packetmode: Ascii | Binary | String Buffer
      mask Callback packetmode: stm32f4_usart_callback('packetmode');
      mask Callback binheader: stm32f4_usart_callback('binheader');
      mask Callback binterminator: stm32f4_usart_callback('binterminator');
      mask Callback porttype_double: stm32f4_usart_callback('porttype');
      mask Callback porttype_single: stm32f4_usart_callback('porttype');
      mask Callback porttype_int8: stm32f4_usart_callback('porttype');
      mask Callback porttype_uint8: stm32f4_usart_callback('porttype');
      mask Callback porttype_int16: stm32f4_usart_callback('porttype');
      mask Callback porttype_uint16: stm32f4_usart_callback('porttype');
      mask Callback porttype_int32: stm32f4_usart_callback('porttype');
      mask Callback porttype_uint32: stm32f4_usart_callback('porttype');
      mask Callback asciiformat: stm32f4_usart_callback('asciiformat');
      mask TypeOptions rx_asciiterminator: CR (0x0D - "\r") | LF (0x0A - "\n") | CRLF (0x0D 0x0A - "\r\n")
      mask Callback rx_asciiterminator: stm32f4_usart_callback('rx_asciiterminator');
      mask TypeOptions tx_asciiterminator: CR (0x0D - "\r") | LF (0x0A - "\n") | CRLF (0x0D 0x0A - "\r\n") | None
      mask Callback tx_asciiterminator: stm32f4_usart_callback('tx_asciiterminator');
      mask TypeOptions storagename: <Please insert a storage name> | S
      mask Callback storagename: stm32f4_usart_callback('storagename');
      mask Callback varname: stm32f4_usart_callback('varname');
      mask Callback sampletime: stm32f4_usart_callback('sampletime');
      mask Callback sampletimestr: stm32f4_usart_callback('sampletimestr');
      mask Callback blockid: stm32f4_usart_callback('blockid');
      mask Display: text(0.95, 0.5, 'Module: USART3_Tx\nPacket: Ascii\nTransfer: Blocking\nTs (sec): -1','ver','middle','hor','right'); port_label('input', 1,'single'); port_label('input', 2,'single'); port_label('input', 3,'single'); port_label('input', 4,'single'); port_label('input', 5,'single'); port_label('input', 6,'single'); port_label('input', 7,'single'); port_label('input', 8,'single'); port_label('input', 9,'single'); port_label('input', 10,'single'); port_label('input', 11,'single'); port_label('input', 12,'single'); port_label('input', 13,'single'); port_label('input', 14,'single'); port_label('input', 15,'single'); port_label('input', 16,'single'); port_label('input', 17,'single'); port_label('input', 18,'single'); port_label('input', 19,'single'); port_label('input', 20,'single'); port_label('input', 21,'single');
  wires:
  In1/1 -> Data Type Conversion22/1, UART Tx1/1
  In4/1 -> Data Type Conversion1/1, Data Type Conversion2/1
  In5/1 -> Data Type Conversion14/1
  Data Store Read/2 -> Data Type Conversion6/1
  Data Store Read/3 -> Data Type Conversion7/1
  Data Type Conversion4/1 -> Data Store Write/1
  MATLAB Function/1(y) -> Data Type Conversion4/1
  Data Type Conversion7/1 -> UART Tx1/8
  Data Type Conversion6/1 -> UART Tx1/7
  Data Store Read/1 -> Data Type Conversion5/1
  Data Type Conversion5/1 -> UART Tx1/6
  Data Store Read/5 -> Data Type Conversion9/1
  Data Store Read/4 -> Data Type Conversion8/1
  Data Store Read/6 -> Data Type Conversion10/1
  Data Store Read/7 -> Data Type Conversion11/1
  Data Store Read/8 -> Data Type Conversion12/1
  Data Type Conversion8/1 -> UART Tx1/9
  Data Type Conversion9/1 -> UART Tx1/10
  Data Type Conversion10/1 -> UART Tx1/11
  Data Type Conversion11/1 -> UART Tx1/12
  Data Type Conversion12/1 -> UART Tx1/13
  Data Store Read/9 -> Data Type Conversion13/1
  Data Type Conversion13/1 -> UART Tx1/14
  Data Type Conversion14/1 -> MATLAB Function/1(u)
  Data Store Read/10 -> Data Type Conversion15/1
  Data Store Read/11 -> Data Type Conversion16/1
  Data Store Read/12 -> Data Type Conversion17/1
  Data Store Read/13 -> Data Type Conversion18/1
  Data Store Read/14 -> Data Type Conversion19/1
  Data Store Read/15 -> Data Type Conversion20/1
  Data Store Read/16 -> Data Type Conversion21/1
  Data Type Conversion15/1 -> UART Tx1/15
  Data Type Conversion16/1 -> UART Tx1/16
  Data Type Conversion17/1 -> UART Tx1/17
  Data Type Conversion18/1 -> UART Tx1/18
  Data Type Conversion20/1 -> UART Tx1/20
  Data Type Conversion21/1 -> UART Tx1/21
  Data Type Conversion19/1 -> UART Tx1/19
  Data Type Conversion22/1 -> Data Store Write1/1
  Data Type Conversion23/1 -> Data Store Write2/1
  In2/1 -> Data Type Conversion23/1, UART Tx1/2
  Data Type Conversion24/1 -> Data Store Write3/1
  In3/1 -> Data Type Conversion24/1, UART Tx1/3
  Constant/1 -> Data Type Conversion3/1
  Data Type Conversion1/1 -> UART Tx1/4
  Data Type Conversion2/1 -> Data Store Write4/1
  Data Type Conversion3/1 -> UART Tx1/5

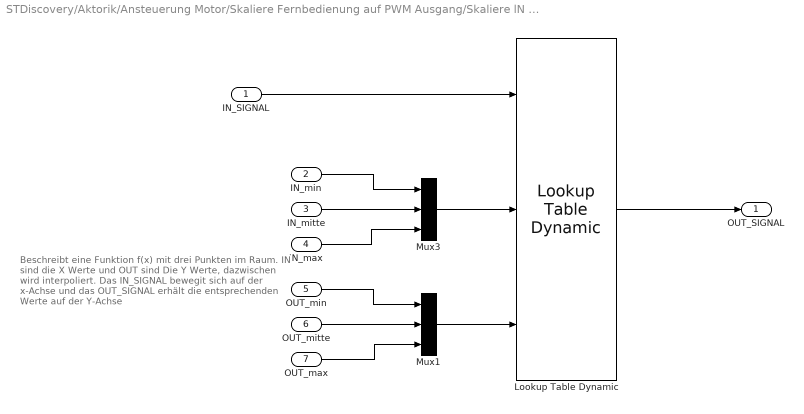
== system STDiscovery/Aktorik/Ansteuerung Motor/Skaliere Fernbedienung auf PWM Ausgang/Skaliere lN nach OUT ==
  note: Beschreibt eine Funktion f(x) mit drei Punkten im Raum.
      | IN sind die X Werte und OUT sind Die Y Werte,
      | dazwischen wird interpoliert.
      |
      | Das IN_SIGNAL bewegit sich auf der x-Achse und
      | das OUT_SIGNAL erhält die entsprechenden Werte auf
      | der Y-Achse
  IN_SIGNAL : Inport
  IN_min : Inport  Port=2
  IN_mitte : Inport  Port=3
  IN_max : Inport  Port=4
  OUT_min : Inport  Port=5
  OUT_mitte : Inport  Port=6
  OUT_max : Inport  Port=7
  Lookup Table Dynamic : simulink/Lookup Tables/Lookup Table Dynamic  LookUpMeth=Interpolation-Use End Values  OutDataType=fixdt('double')  OutScaling=[]  OutputDataTypeScalingMode=Specify via dialog  OutDataTypeStr=fixdt('double')  DoSatur=off
      settings: SourceProductName=Simulink
  Mux1 : Mux  Inputs=3
  Mux3 : Mux  Inputs=3
  OUT_SIGNAL : Outport
  wires:
  IN_SIGNAL/1 -> Lookup Table Dynamic/1
  IN_max/1 -> Mux3/3
  IN_mitte/1 -> Mux3/2
  IN_min/1 -> Mux3/1
  OUT_min/1 -> Mux1/1
  OUT_mitte/1 -> Mux1/2
  OUT_max/1 -> Mux1/3
  Lookup Table Dynamic/1 -> OUT_SIGNAL/1
  Mux1/1 -> Lookup Table Dynamic/3
  Mux3/1 -> Lookup Table Dynamic/2

== system STDiscovery/Aktorik/Ansteuerung Motor/Skaliere Jetson( + -100) auf PWM Ausgang/Skaliere lN nach OUT ==
  note: Beschreibt eine Funktion f(x) mit drei Punkten im Raum.
      | IN sind die X Werte und OUT sind Die Y Werte,
      | dazwischen wird interpoliert.
      |
      | Das IN_SIGNAL bewegit sich auf der x-Achse und
      | das OUT_SIGNAL erhält die entsprechenden Werte auf
      | der Y-Achse
  IN_SIGNAL : Inport
  IN_min : Inport  Port=2
  IN_mitte : Inport  Port=3
  IN_max : Inport  Port=4
  OUT_min : Inport  Port=5
  OUT_mitte : Inport  Port=6
  OUT_max : Inport  Port=7
  Lookup Table Dynamic : simulink/Lookup Tables/Lookup Table Dynamic  LookUpMeth=Interpolation-Use End Values  OutDataType=fixdt('double')  OutScaling=[]  OutputDataTypeScalingMode=Specify via dialog  OutDataTypeStr=fixdt('double')  DoSatur=off
      settings: SourceProductName=Simulink
  Mux1 : Mux  Inputs=3
  Mux3 : Mux  Inputs=3
  OUT_SIGNAL : Outport
  wires:
  IN_SIGNAL/1 -> Lookup Table Dynamic/1
  IN_max/1 -> Mux3/3
  IN_mitte/1 -> Mux3/2
  IN_min/1 -> Mux3/1
  OUT_min/1 -> Mux1/1
  OUT_mitte/1 -> Mux1/2
  OUT_max/1 -> Mux1/3
  Lookup Table Dynamic/1 -> OUT_SIGNAL/1
  Mux1/1 -> Lookup Table Dynamic/3
  Mux3/1 -> Lookup Table Dynamic/2

== system STDiscovery/Aktorik/Ansteuerung Motor/Skaliere PWM Ausgang wieder in wert zwischen( + -100) zum Loggen /Skaliere lN nach OUT ==
  note: Beschreibt eine Funktion f(x) mit drei Punkten im Raum.
      | IN sind die X Werte und OUT sind Die Y Werte,
      | dazwischen wird interpoliert.
      |
      | Das IN_SIGNAL bewegit sich auf der x-Achse und
      | das OUT_SIGNAL erhält die entsprechenden Werte auf
      | der Y-Achse
  IN_SIGNAL : Inport
  IN_min : Inport  Port=2
  IN_mitte : Inport  Port=3
  IN_max : Inport  Port=4
  OUT_min : Inport  Port=5
  OUT_mitte : Inport  Port=6
  OUT_max : Inport  Port=7
  Lookup Table Dynamic : simulink/Lookup Tables/Lookup Table Dynamic  LookUpMeth=Interpolation-Use End Values  OutDataType=fixdt('double')  OutScaling=[]  OutputDataTypeScalingMode=Specify via dialog  OutDataTypeStr=fixdt('double')  DoSatur=off
      settings: SourceProductName=Simulink
  Mux1 : Mux  Inputs=3
  Mux3 : Mux  Inputs=3
  OUT_SIGNAL : Outport
  wires:
  IN_SIGNAL/1 -> Lookup Table Dynamic/1
  IN_max/1 -> Mux3/3
  IN_mitte/1 -> Mux3/2
  IN_min/1 -> Mux3/1
  OUT_min/1 -> Mux1/1
  OUT_mitte/1 -> Mux1/2
  OUT_max/1 -> Mux1/3
  Lookup Table Dynamic/1 -> OUT_SIGNAL/1
  Mux1/1 -> Lookup Table Dynamic/3
  Mux3/1 -> Lookup Table Dynamic/2

== system STDiscovery/Aktorik/Ansteuerung Servo/Skaliere Fernbedienung auf PWM Ausgang/Skaliere lN nach OUT ==
  note: Beschreibt eine Funktion f(x) mit drei Punkten im Raum.
      | IN sind die X Werte und OUT sind Die Y Werte,
      | dazwischen wird interpoliert.
      |
      | Das IN_SIGNAL bewegit sich auf der x-Achse und
      | das OUT_SIGNAL erhält die entsprechenden Werte auf
      | der Y-Achse
  IN_SIGNAL : Inport
  IN_min : Inport  Port=2
  IN_mitte : Inport  Port=3
  IN_max : Inport  Port=4
  OUT_min : Inport  Port=5
  OUT_mitte : Inport  Port=6
  OUT_max : Inport  Port=7
  Lookup Table Dynamic : simulink/Lookup Tables/Lookup Table Dynamic  LookUpMeth=Interpolation-Use End Values  OutDataType=fixdt('double')  OutScaling=[]  OutputDataTypeScalingMode=Specify via dialog  OutDataTypeStr=fixdt('double')  DoSatur=off
      settings: SourceProductName=Simulink
  Mux1 : Mux  Inputs=3
  Mux3 : Mux  Inputs=3
  OUT_SIGNAL : Outport
  wires:
  IN_SIGNAL/1 -> Lookup Table Dynamic/1
  IN_max/1 -> Mux3/3
  IN_mitte/1 -> Mux3/2
  IN_min/1 -> Mux3/1
  OUT_min/1 -> Mux1/1
  OUT_mitte/1 -> Mux1/2
  OUT_max/1 -> Mux1/3
  Lookup Table Dynamic/1 -> OUT_SIGNAL/1
  Mux1/1 -> Lookup Table Dynamic/3
  Mux3/1 -> Lookup Table Dynamic/2

== system STDiscovery/Aktorik/Ansteuerung Servo/Skaliere Stellwinkel auf PWM Ausgang/Skaliere lN nach OUT ==
  note: Beschreibt eine Funktion f(x) mit drei Punkten im Raum.
      | IN sind die X Werte und OUT sind Die Y Werte,
      | dazwischen wird interpoliert.
      |
      | Das IN_SIGNAL bewegit sich auf der x-Achse und
      | das OUT_SIGNAL erhält die entsprechenden Werte auf
      | der Y-Achse
  IN_SIGNAL : Inport
  IN_min : Inport  Port=2
  IN_mitte : Inport  Port=3
  IN_max : Inport  Port=4
  OUT_min : Inport  Port=5
  OUT_mitte : Inport  Port=6
  OUT_max : Inport  Port=7
  Lookup Table Dynamic : simulink/Lookup Tables/Lookup Table Dynamic  LookUpMeth=Interpolation-Use End Values  OutDataType=fixdt('double')  OutScaling=[]  OutputDataTypeScalingMode=Specify via dialog  OutDataTypeStr=fixdt('double')  DoSatur=off
      settings: SourceProductName=Simulink
  Mux1 : Mux  Inputs=3
  Mux3 : Mux  Inputs=3
  OUT_SIGNAL : Outport
  wires:
  IN_SIGNAL/1 -> Lookup Table Dynamic/1
  IN_max/1 -> Mux3/3
  IN_mitte/1 -> Mux3/2
  IN_min/1 -> Mux3/1
  OUT_min/1 -> Mux1/1
  OUT_mitte/1 -> Mux1/2
  OUT_max/1 -> Mux1/3
  Lookup Table Dynamic/1 -> OUT_SIGNAL/1
  Mux1/1 -> Lookup Table Dynamic/3
  Mux3/1 -> Lookup Table Dynamic/2

== system STDiscovery/Aktorik/Ansteuerung Servo/Skaliere steuer Stellwinkel wieder in Grad zum Loggen/Skaliere lN nach OUT ==
  note: Beschreibt eine Funktion f(x) mit drei Punkten im Raum.
      | IN sind die X Werte und OUT sind Die Y Werte,
      | dazwischen wird interpoliert.
      |
      | Das IN_SIGNAL bewegit sich auf der x-Achse und
      | das OUT_SIGNAL erhält die entsprechenden Werte auf
      | der Y-Achse
  IN_SIGNAL : Inport
  IN_min : Inport  Port=2
  IN_mitte : Inport  Port=3
  IN_max : Inport  Port=4
  OUT_min : Inport  Port=5
  OUT_mitte : Inport  Port=6
  OUT_max : Inport  Port=7
  Lookup Table Dynamic : simulink/Lookup Tables/Lookup Table Dynamic  LookUpMeth=Interpolation-Use End Values  OutDataType=fixdt('double')  OutScaling=[]  OutputDataTypeScalingMode=Specify via dialog  OutDataTypeStr=fixdt('double')  DoSatur=off
      settings: SourceProductName=Simulink
  Mux1 : Mux  Inputs=3
  Mux3 : Mux  Inputs=3
  OUT_SIGNAL : Outport
  wires:
  IN_SIGNAL/1 -> Lookup Table Dynamic/1
  IN_max/1 -> Mux3/3
  IN_mitte/1 -> Mux3/2
  IN_min/1 -> Mux3/1
  OUT_min/1 -> Mux1/1
  OUT_mitte/1 -> Mux1/2
  OUT_max/1 -> Mux1/3
  Lookup Table Dynamic/1 -> OUT_SIGNAL/1
  Mux1/1 -> Lookup Table Dynamic/3
  Mux3/1 -> Lookup Table Dynamic/2

== matlab function STDiscovery/Kommunikation/vom Jetson empfangen //// ST zu Debug PC /Subsystem3/MATLAB Function ==
  data: u input; y output
function y = fcn(u)
y =de2bi( u, 32 );

== matlab function STDiscovery/Aktorik/Ansteuerung Servo/MATLAB Function ==
  data: Meter_Lookahead_Distance input; Phi_stell output; AbweichungVonMitte input; MomentanGeschwindigkeit input; Phi_current input
function Phi_stell  = Path_Follower (Meter_Lookahead_Distance, AbweichungVonMitte, MomentanGeschwindigkeit, Phi_current)


if MomentanGeschwindigkeit==0
MomentanGeschwindigkeit=0.01    
end


if isnan(Phi_current)
    Phi_current=0
end

Radstand=0.27 %ToDo 27cm Radbreite: 15,7cm
c_ref=(2*AbweichungVonMitte) / (Meter_Lookahead_Distance^2) %gewünschte Kurve
w_ref= MomentanGeschwindigkeit*c_ref %gewünschte Rotationsgeschwindigkeit
w_current= MomentanGeschwindigkeit*(tan(Phi_current)/Radstand) %momentane Rotationsgeschwindigkeit

e=w_ref-w_current %Abweichung aktuelle Winkelgeschwindigkeit zu gewünschter


Phi_stell=rad2deg(atan((e*Radstand)/MomentanGeschwindigkeit))
     %   e=rad2deg(atan((e*Radstand)/MomentanGeschwindigkeit)) %Umrechnung Winkelgeschwindigkeit in stellwinkel
    
if isnan(Phi_stell)
Phi_stell=0
end


end

== matlab function STDiscovery/Kommunikation/sende an Jetson zurueck //// ST zu Debug PC /Subsystem3/MATLAB Function1 ==
  data: u input; y output
function y = fcn(u)
y=bi2de(u');

== matlab function STDiscovery/MomentangeschwindigkeitEinlesen/MATLAB Function ==
  data: x input; y output
function y = fcn(x)

y = 0.0158*x;
